simulink model "Simulation"  (R2016a)
settings: Solver=FixedStepAuto  StartTime=0.0  StopTime=20  FixedStep=0.01  RelTol=1e-3
undefined symbols (not defined in the file or in its folder): beta, g0, g1, g2, g3, gamma, kappa, landa, nu
(part 29 of 30)

== matlab function Simulation/U ==
  data: Ueq input; Uas input; u1 output; theta input; thetadot input; u2 output; u3 output; u4 output; u5 output; u6 output
function [u1,u2,u3,u4,u5,u6] = fcn(Ueq,Uas,theta,thetadot)


theta1=theta(1)
theta2=theta(2)
theta3=theta(3)
theta4=theta(4)
theta5=theta(5)
theta6=theta(6)

thetadot1=thetadot(1)
thetadot2=thetadot(2)
thetadot3=thetadot(3)
thetadot4=thetadot(4)
thetadot5=thetadot(5)
thetadot6=thetadot(6)
MM=[ 0.1*cos(theta2 + theta3)^2 + (0.1*cos(theta2)*cos(theta3)*cos(theta6)*sin(theta4) - 0.1*cos(theta6)*sin(theta2)*sin(theta3)*sin(theta4) + 0.1*cos(theta2)*sin(theta3)*sin(theta5)*sin(theta6) + 0.1*cos(theta3)*sin(theta2)*sin(theta5)*sin(theta6) - 0.1*cos(theta2)*cos(theta3)*cos(theta4)*cos(theta5)*sin(theta6) + 0.1*cos(theta4)*cos(theta5)*sin(theta2)*sin(theta3)*sin(theta6))*(cos(theta2)*cos(theta3)*cos(theta6)*sin(theta4) - 1.0*cos(theta6)*sin(theta2)*sin(theta3)*sin(theta4) + cos(theta2)*sin(theta3)*sin(theta5)*sin(theta6) + cos(theta3)*sin(theta2)*sin(theta5)*sin(theta6) - 1.0*cos(theta2)*cos(theta3)*cos(theta4)*cos(theta5)*sin(theta6) + cos(theta4)*cos(theta5)*sin(theta2)*sin(theta3)*sin(theta6)) + 0.2*sin(theta2 + theta3)^2 + (0.2*cos(theta2)*sin(theta4)*sin(theta5) + 0.4*sin(theta2)*sin(theta3)*sin(theta4) - 0.4*cos(theta2)*cos(theta3)*sin(theta4) + 0.4*cos(theta2)*cos(theta3)*cos(theta6)*sin(theta4) + 0.4*cos(theta2)*cos(theta3)*sin(theta4)*sin(theta5) - 0.4*cos(theta6)*sin(theta2)*sin(theta3)*sin(theta4) + 0.4*cos(theta2)*sin(theta3)*sin(theta5)*sin(theta6) + 0.4*cos(theta3)*sin(theta2)*sin(theta5)*sin(theta6) - 0.4*sin(theta2)*sin(theta3)*sin(theta4)*sin(theta5) - 0.4*cos(theta2)*cos(theta3)*cos(theta4)*cos(theta5)*sin(theta6) + 0.4*cos(theta4)*cos(theta5)*sin(theta2)*sin(theta3)*sin(theta6))^2 + 0.14*cos(theta2)^2 + 0.1*sin(theta2)^2 + (cos(theta2)*sin(theta3)*sin(theta5) + cos(theta3)*sin(theta2)*sin(theta5) - 1.0*cos(theta2)*cos(theta3)*cos(theta4)*cos(theta5) + cos(theta4)*cos(theta5)*sin(theta2)*sin(theta3))*(0.1*cos(theta2)*sin(theta3)*sin(theta5) + 0.1*cos(theta3)*sin(theta2)*sin(theta5) - 0.1*cos(theta2)*cos(theta3)*cos(theta4)*cos(theta5) + 0.1*cos(theta4)*cos(theta5)*sin(theta2)*sin(theta3)) + 2.0*(cos(theta2)*cos(theta5)*sin(theta3) + cos(theta3)*cos(theta5)*sin(theta2) + cos(theta2)*cos(theta3)*cos(theta4)*sin(theta5) - 1.0*cos(theta4)*sin(theta2)*sin(theta3)*sin(theta5))*(0.1*cos(theta2)*cos(theta5)*sin(theta3) + 0.1*cos(theta3)*cos(theta5)*sin(theta2) + 0.1*cos(theta2)*cos(theta3)*cos(theta4)*sin(theta5) - 0.1*cos(theta4)*sin(theta2)*sin(theta3)*sin(theta5)) + 0.04*cos(theta4)^2*(2.0*cos(theta2 + theta3) + cos(theta2))^2 + 0.1*cos(theta2 + theta3)^2*cos(theta4)^2 + 0.2*cos(theta2 + theta3)^2*sin(theta4)^2 + (0.1*cos(theta2)*cos(theta6)*sin(theta3)*sin(theta5) - 0.1*cos(theta2)*cos(theta3)*sin(theta4)*sin(theta6) + 0.1*cos(theta3)*cos(theta6)*sin(theta2)*sin(theta5) + 0.1*sin(theta2)*sin(theta3)*sin(theta4)*sin(theta6) - 0.1*cos(theta2)*cos(theta3)*cos(theta4)*cos(theta5)*cos(theta6) + 0.1*cos(theta4)*cos(theta5)*cos(theta6)*sin(theta2)*sin(theta3))*(cos(theta2)*cos(theta6)*sin(theta3)*sin(theta5) - 1.0*cos(theta2)*cos(theta3)*sin(theta4)*sin(theta6) + cos(theta3)*cos(theta6)*sin(theta2)*sin(theta5) + sin(theta2)*sin(theta3)*sin(theta4)*sin(theta6) - 1.0*cos(theta2)*cos(theta3)*cos(theta4)*cos(theta5)*cos(theta6) + cos(theta4)*cos(theta5)*cos(theta6)*sin(theta2)*sin(theta3)) + 0.04*cos(theta4)^2*(cos(theta2 + theta3) + cos(theta2))^2 + 0.04*sin(theta4)^2*(cos(theta2 + theta3) + cos(theta2))^2 + (0.2*cos(theta2)*cos(theta5)*cos(theta6)*sin(theta4) - 0.4*cos(theta2)*cos(theta3)*cos(theta4)*sin(theta6) - 0.2*cos(theta2)*cos(theta4)*sin(theta6) + 0.4*cos(theta2)*cos(theta5)*sin(theta3)*sin(theta6) + 0.4*cos(theta3)*cos(theta5)*sin(theta2)*sin(theta6) + 0.4*cos(theta4)*sin(theta2)*sin(theta3)*sin(theta6) + 0.4*cos(theta2)*cos(theta3)*cos(theta5)*cos(theta6)*sin(theta4) + 0.4*cos(theta2)*cos(theta3)*cos(theta4)*sin(theta5)*sin(theta6) - 0.4*cos(theta5)*cos(theta6)*sin(theta2)*sin(theta3)*sin(theta4) - 0.4*cos(theta4)*sin(theta2)*sin(theta3)*sin(theta5)*sin(theta6))^2 + (0.2*cos(theta2)*cos(theta4)*cos(theta6) + 0.4*cos(theta2)*cos(theta5)*sin(theta3) + 0.4*cos(theta3)*cos(theta5)*sin(theta2) + 0.4*cos(theta2)*cos(theta3)*cos(theta4)*cos(theta6) + 0.4*cos(theta2)*cos(theta3)*cos(theta4)*sin(theta5) - 0.4*cos(theta2)*cos(theta5)*cos(theta6)*sin(theta3) - 0.4*cos(theta3)*cos(theta5)*cos(theta6)*sin(theta2) - 0.4*cos(theta4)*cos(theta6)*sin(theta2)*sin(theta3) + 0.2*cos(theta2)*cos(theta5)*sin(theta4)*sin(theta6) - 0.4*cos(theta4)*sin(theta2)*sin(theta3)*sin(theta5) - 0.4*cos(theta2)*cos(theta3)*cos(theta4)*cos(theta6)*sin(theta5) + 0.4*cos(theta2)*cos(theta3)*cos(theta5)*sin(theta4)*sin(theta6) + 0.4*cos(theta4)*cos(theta6)*sin(theta2)*sin(theta3)*sin(theta5) - 0.4*cos(theta5)*sin(theta2)*sin(theta3)*sin(theta4)*sin(theta6))^2 + 0.04*cos(theta5)^2*sin(theta4)^2*(2.0*cos(theta2 + theta3) + cos(theta2))^2 + 0.04*sin(theta4)^2*sin(theta5)^2*(2.0*cos(theta2 + theta3) + cos(theta2))^2 + 0.1, 0.16*cos(theta2)*cos(theta3)*cos(theta4)*sin(theta4) - 0.08*cos(theta4)*sin(theta2)*sin(theta6) - 0.08*cos(theta5)*sin(theta2)*sin(theta4) + 0.16*cos(theta2)*cos(theta3)*cos(theta5)*sin(theta6) - 0.16*cos(theta2)*cos(theta5)*sin(theta3)*sin(theta4) - 0.16*cos(theta3)*cos(theta5)*sin(theta2)*sin(theta4) - 0.16*cos(theta2)*cos(theta4)*sin(theta3)*sin(theta6) - 0.16*cos(theta3)*cos(theta4)*sin(theta2)*sin(theta6) + 0.08*cos(theta5)*cos(theta6)*sin(theta2)*sin(theta4) - 0.16*cos(theta4)*sin(theta2)*sin(theta3)*sin(theta4) - 0.16*cos(theta5)*sin(theta2)*sin(theta3)*sin(theta6) - 0.16*cos(theta2)*cos(theta3)*cos(theta4)*cos(theta5)^2*sin(theta4) - 0.16*cos(theta2)*cos(theta3)*cos(theta4)*cos(theta6)^2*sin(theta4) - 0.32*cos(theta2)*cos(theta3)*cos(theta4)^2*cos(theta5)*sin(theta6) + 0.16*cos(theta4)*cos(theta5)^2*sin(theta2)*sin(theta3)*sin(theta4) + 0.16*cos(theta4)*cos(theta6)^2*sin(theta2)*sin(theta3)*sin(theta4) + 0.32*cos(theta4)^2*cos(theta5)*sin(theta2)*sin(theta3)*sin(theta6) - 0.16*cos(theta2)*cos(theta3)*cos(theta5)*cos(theta6)*sin(theta6) + 0.16*cos(theta2)*cos(theta5)*cos(theta6)*sin(theta3)*sin(theta4) + 0.16*cos(theta3)*cos(theta5)*cos(theta6)*sin(theta2)*sin(theta4) + 0.16*cos(theta2)*cos(theta5)*sin(theta3)*sin(theta4)*sin(theta5) + 0.16*cos(theta3)*cos(theta5)*sin(theta2)*sin(theta4)*sin(theta5) + 0.16*cos(theta2)*cos(theta4)*sin(theta3)*sin(theta5)*sin(theta6) + 0.16*cos(theta3)*cos(theta4)*sin(theta2)*sin(theta5)*sin(theta6) + 0.16*cos(theta5)*cos(theta6)*sin(theta2)*sin(theta3)*sin(theta6) - 0.16*cos(theta2)*cos(theta3)*cos(theta4)*cos(theta5)^2*cos(theta6)^2*sin(theta4) + 0.16*cos(theta4)*cos(theta5)^2*cos(theta6)^2*sin(theta2)*sin(theta3)*sin(theta4) - 0.32*cos(theta2)*cos(theta5)*cos(theta6)*sin(theta3)*sin(theta4)*sin(theta5) - 0.32*cos(theta3)*cos(theta5)*cos(theta6)*sin(theta2)*sin(theta4)*sin(theta5) - 0.16*cos(theta2)*cos(theta4)*cos(theta6)*sin(theta3)*sin(theta5)*sin(theta6) - 0.16*cos(theta3)*cos(theta4)*cos(theta6)*sin(theta2)*sin(theta5)*sin(theta6) + 0.32*cos(theta2)*cos(theta3)*cos(theta4)*cos(theta5)^2*cos(theta6)*sin(theta4) + 0.32*cos(theta2)*cos(theta3)*cos(theta4)^2*cos(theta5)*cos(theta6)*sin(theta6) - 0.32*cos(theta4)*cos(theta5)^2*cos(theta6)*sin(theta2)*sin(theta3)*sin(theta4) + 0.16*cos(theta2)*cos(theta5)*cos(theta6)^2*sin(theta3)*sin(theta4)*sin(theta5) + 0.16*cos(theta3)*cos(theta5)*cos(theta6)^2*sin(theta2)*sin(theta4)*sin(theta5) - 0.32*cos(theta4)^2*cos(theta5)*cos(theta6)*sin(theta2)*sin(theta3)*sin(theta6), 0.16*cos(theta2)*cos(theta3)*cos(theta4)*sin(theta4) + 0.16*cos(theta2)*cos(theta3)*cos(theta5)*sin(theta6) - 0.16*cos(theta2)*cos(theta5)*sin(theta3)*sin(theta4) - 0.16*cos(theta3)*cos(theta5)*sin(theta2)*sin(theta4) - 0.16*cos(theta2)*cos(theta4)*sin(theta3)*sin(theta6) - 0.16*cos(theta3)*cos(theta4)*sin(theta2)*sin(theta6) - 0.16*cos(theta4)*sin(theta2)*sin(theta3)*sin(theta4) - 0.16*cos(theta5)*sin(theta2)*sin(theta3)*sin(theta6) - 0.16*cos(theta2)*cos(theta3)*cos(theta4)*cos(theta5)^2*sin(theta4) - 0.16*cos(theta2)*cos(theta3)*cos(theta4)*cos(theta6)^2*sin(theta4) - 0.32*cos(theta2)*cos(theta3)*cos(theta4)^2*cos(theta5)*sin(theta6) + 0.16*cos(theta4)*cos(theta5)^2*sin(theta2)*sin(theta3)*sin(theta4) + 0.16*cos(theta4)*cos(theta6)^2*sin(theta2)*sin(theta3)*sin(theta4) + 0.32*cos(theta4)^2*cos(theta5)*sin(theta2)*sin(theta3)*sin(theta6) - 0.16*cos(theta2)*cos(theta3)*cos(theta5)*cos(theta6)*sin(theta6) + 0.16*cos(theta2)*cos(theta5)*cos(theta6)*sin(theta3)*sin(theta4) + 0.16*cos(theta3)*cos(theta5)*cos(theta6)*sin(theta2)*sin(theta4) + 0.16*cos(theta2)*cos(theta5)*sin(theta3)*sin(theta4)*sin(theta5) + 0.16*cos(theta3)*cos(theta5)*sin(theta2)*sin(theta4)*sin(theta5) + 0.16*cos(theta2)*cos(theta4)*sin(theta3)*sin(theta5)*sin(theta6) + 0.16*cos(theta3)*cos(theta4)*sin(theta2)*sin(theta5)*sin(theta6) + 0.16*cos(theta5)*cos(theta6)*sin(theta2)*sin(theta3)*sin(theta6) - 0.16*cos(theta2)*cos(theta3)*cos(theta4)*cos(theta5)^2*cos(theta6)^2*sin(theta4) + 0.16*cos(theta4)*cos(theta5)^2*cos(theta6)^2*sin(theta2)*sin(theta3)*sin(theta4) - 0.32*cos(theta2)*cos(theta5)*cos(theta6)*sin(theta3)*sin(theta4)*sin(theta5) - 0.32*cos(theta3)*cos(theta5)*cos(theta6)*sin(theta2)*sin(theta4)*sin(theta5) - 0.16*cos(theta2)*cos(theta4)*cos(theta6)*sin(theta3)*sin(theta5)*sin(theta6) - 0.16*cos(theta3)*cos(theta4)*cos(theta6)*sin(theta2)*sin(theta5)*sin(theta6) + 0.32*cos(theta2)*cos(theta3)*cos(theta4)*cos(theta5)^2*cos(theta6)*sin(theta4) + 0.32*cos(theta2)*cos(theta3)*cos(theta4)^2*cos(theta5)*cos(theta6)*sin(theta6) - 0.32*cos(theta4)*cos(theta5)^2*cos(theta6)*sin(theta2)*sin(theta3)*sin(theta4) + 0.16*cos(theta2)*cos(theta5)*cos(theta6)^2*sin(theta3)*sin(theta4)*sin(theta5) + 0.16*cos(theta3)*cos(theta5)*cos(theta6)^2*sin(theta2)*sin(theta4)*sin(theta5) - 0.32*cos(theta4)^2*cos(theta5)*cos(theta6)*sin(theta2)*sin(theta3)*sin(theta6), 0.46*cos(theta2)*sin(theta3) + 0.46*cos(theta3)*sin(theta2) + 0.08*cos(theta2)*sin(theta4)*sin(theta6) + 0.16*cos(theta2)*cos(theta5)^2*sin(theta3) + 0.16*cos(theta3)*cos(theta5)^2*sin(theta2) - 0.16*cos(theta2)*cos(theta6)^2*sin(theta3) - 0.16*cos(theta3)*cos(theta6)^2*sin(theta2) - 0.08*cos(theta2)*cos(theta4)*cos(theta5) - 0.32*cos(theta2)*cos(theta5)^2*cos(theta6)*sin(theta3) - 0.32*cos(theta3)*cos(theta5)^2*cos(theta6)*sin(theta2) + 0.16*cos(theta2)*cos(theta5)^2*cos(theta6)^2*sin(theta3) + 0.16*cos(theta3)*cos(theta5)^2*cos(theta6)^2*sin(theta2) - 0.16*cos(theta2)*cos(theta3)*cos(theta4)*cos(theta5) + 0.08*cos(theta2)*cos(theta4)*cos(theta5)*cos(theta6) + 0.16*cos(theta4)*cos(theta5)*sin(theta2)*sin(theta3) + 0.16*cos(theta2)*cos(theta3)*sin(theta4)*sin(theta6) - 0.16*sin(theta2)*sin(theta3)*sin(theta4)*sin(theta6) + 0.16*cos(theta2)*cos(theta3)*cos(theta4)*cos(theta5)*cos(theta6) + 0.16*cos(theta2)*cos(theta3)*cos(theta4)*cos(theta5)*sin(theta5) - 0.16*cos(theta4)*cos(theta5)*cos(theta6)*sin(theta2)*sin(theta3) - 0.16*cos(theta4)*cos(theta5)*sin(theta2)*sin(theta3)*sin(theta5) - 0.16*cos(theta2)*cos(theta3)*sin(theta4)*sin(theta5)*sin(theta6) + 0.16*sin(theta2)*sin(theta3)*sin(theta4)*sin(theta5)*sin(theta6) - 0.32*cos(theta2)*cos(theta3)*cos(theta4)*cos(theta5)*cos(theta6)*sin(theta5) + 0.32*cos(theta4)*cos(theta5)*cos(theta6)*sin(theta2)*sin(theta3)*sin(theta5) + 0.16*cos(theta2)*cos(theta3)*cos(theta6)*sin(theta4)*sin(theta5)*sin(theta6) - 0.16*cos(theta6)*sin(theta2)*sin(theta3)*sin(theta4)*sin(theta5)*sin(theta6) + 0.16*cos(theta2)*cos(theta3)*cos(theta4)*cos(theta5)*cos(theta6)^2*sin(theta5) - 0.16*cos(theta4)*cos(theta5)*cos(theta6)^2*sin(theta2)*sin(theta3)*sin(theta5), 0.08*cos(theta2)*sin(theta4)*sin(theta5) + 0.36*sin(theta2)*sin(theta3)*sin(theta4) - 0.36*cos(theta2)*cos(theta3)*sin(theta4) - 0.16*cos(theta2)*cos(theta3)*cos(theta6)^2*sin(theta4) + 0.16*cos(theta6)^2*sin(theta2)*sin(theta3)*sin(theta4) + 0.32*cos(theta2)*cos(theta3)*cos(theta6)*sin(theta4) + 0.16*cos(theta2)*cos(theta3)*sin(theta4)*sin(theta5) - 0.08*cos(theta2)*cos(theta6)*sin(theta4)*sin(theta5) - 0.32*cos(theta6)*sin(theta2)*sin(theta3)*sin(theta4) + 0.16*cos(theta2)*sin(theta3)*sin(theta5)*sin(theta6) + 0.16*cos(theta3)*sin(theta2)*sin(theta5)*sin(theta6) - 0.16*sin(theta2)*sin(theta3)*sin(theta4)*sin(theta5) - 0.16*cos(theta2)*cos(theta3)*cos(theta4)*cos(theta5)*sin(theta6) - 0.16*cos(theta2)*cos(theta3)*cos(theta6)*sin(theta4)*sin(theta5) + 0.16*cos(theta4)*cos(theta5)*sin(theta2)*sin(theta3)*sin(theta6) - 0.16*cos(theta2)*cos(theta6)*sin(theta3)*sin(theta5)*sin(theta6) - 0.16*cos(theta3)*cos(theta6)*sin(theta2)*sin(theta5)*sin(theta6) + 0.16*cos(theta6)*sin(theta2)*sin(theta3)*sin(theta4)*sin(theta5) + 0.16*cos(theta2)*cos(theta3)*cos(theta4)*cos(theta5)*cos(theta6)*sin(theta6) - 0.16*cos(theta4)*cos(theta5)*cos(theta6)*sin(theta2)*sin(theta3)*sin(theta6), 0.08*cos(theta2)*cos(theta4)*cos(theta6) + 0.26*cos(theta2)*cos(theta5)*sin(theta3) + 0.26*cos(theta3)*cos(theta5)*sin(theta2) + 0.16*cos(theta2)*cos(theta3)*cos(theta4)*cos(theta6) + 0.26*cos(theta2)*cos(theta3)*cos(theta4)*sin(theta5) - 0.16*cos(theta2)*cos(theta5)*cos(theta6)*sin(theta3) - 0.16*cos(theta3)*cos(theta5)*cos(theta6)*sin(theta2) - 0.16*cos(theta4)*cos(theta6)*sin(theta2)*sin(theta3) + 0.08*cos(theta2)*cos(theta5)*sin(theta4)*sin(theta6) - 0.26*cos(theta4)*sin(theta2)*sin(theta3)*sin(theta5) - 0.16*cos(theta2)*cos(theta3)*cos(theta4)*cos(theta6)*sin(theta5) + 0.16*cos(theta2)*cos(theta3)*cos(theta5)*sin(theta4)*sin(theta6) + 0.16*cos(theta4)*cos(theta6)*sin(theta2)*sin(theta3)*sin(theta5) - 0.16*cos(theta5)*sin(theta2)*sin(theta3)*sin(theta4)*sin(theta6);
                                                                                                                                                                                                                                                                                                                                                                                                                                                                                                                                                                                                                                                                                                                                                                                                                                                                                                                                                                                                                                                                                                                                                                                                                                                                                                                                                                                                                                                                                                                                                                                                                                                                                                                                                                                                                                                                                                                                                                                                                                                                                                                                                                       0.16*cos(theta2)*cos(theta3)*cos(theta4)*sin(theta4) - 0.08*cos(theta4)*sin(theta2)*sin(theta6) - 0.08*cos(theta5)*sin(theta2)*sin(theta4) + 0.16*cos(theta2)*cos(theta3)*cos(theta5)*sin(theta6) - 0.16*cos(theta2)*cos(theta5)*sin(theta3)*sin(theta4) - 0.16*cos(theta3)*cos(theta5)*sin(theta2)*sin(theta4) - 0.16*cos(theta2)*cos(theta4)*sin(theta3)*sin(theta6) - 0.16*cos(theta3)*cos(theta4)*sin(theta2)*sin(theta6) + 0.08*cos(theta5)*cos(theta6)*sin(theta2)*sin(theta4) - 0.16*cos(theta4)*sin(theta2)*sin(theta3)*sin(theta4) - 0.16*cos(theta5)*sin(theta2)*sin(theta3)*sin(theta6) - 0.16*cos(theta2)*cos(theta3)*cos(theta4)*cos(theta5)^2*sin(theta4) - 0.16*cos(theta2)*cos(theta3)*cos(theta4)*cos(theta6)^2*sin(theta4) - 0.32*cos(theta2)*cos(theta3)*cos(theta4)^2*cos(theta5)*sin(theta6) + 0.16*cos(theta4)*cos(theta5)^2*sin(theta2)*sin(theta3)*sin(theta4) + 0.16*cos(theta4)*cos(theta6)^2*sin(theta2)*sin(theta3)*sin(theta4) + 0.32*cos(theta4)^2*cos(theta5)*sin(theta2)*sin(theta3)*sin(theta6) - 0.16*cos(theta2)*cos(theta3)*cos(theta5)*cos(theta6)*sin(theta6) + 0.16*cos(theta2)*cos(theta5)*cos(theta6)*sin(theta3)*sin(theta4) + 0.16*cos(theta3)*cos(theta5)*cos(theta6)*sin(theta2)*sin(theta4) + 0.16*cos(theta2)*cos(theta5)*sin(theta3)*sin(theta4)*sin(theta5) + 0.16*cos(theta3)*cos(theta5)*sin(theta2)*sin(theta4)*sin(theta5) + 0.16*cos(theta2)*cos(theta4)*sin(theta3)*sin(theta5)*sin(theta6) + 0.16*cos(theta3)*cos(theta4)*sin(theta2)*sin(theta5)*sin(theta6) + 0.16*cos(theta5)*cos(theta6)*sin(theta2)*sin(theta3)*sin(theta6) - 0.16*cos(theta2)*cos(theta3)*cos(theta4)*cos(theta5)^2*cos(theta6)^2*sin(theta4) + 0.16*cos(theta4)*cos(theta5)^2*cos(theta6)^2*sin(theta2)*sin(theta3)*sin(theta4) - 0.32*cos(theta2)*cos(theta5)*cos(theta6)*sin(theta3)*sin(theta4)*sin(theta5) - 0.32*cos(theta3)*cos(theta5)*cos(theta6)*sin(theta2)*sin(theta4)*sin(theta5) - 0.16*cos(theta2)*cos(theta4)*cos(theta6)*sin(theta3)*sin(theta5)*sin(theta6) - 0.16*cos(theta3)*cos(theta4)*cos(theta6)*sin(theta2)*sin(theta5)*sin(theta6) + 0.32*cos(theta2)*cos(theta3)*cos(theta4)*cos(theta5)^2*cos(theta6)*sin(theta4) + 0.32*cos(theta2)*cos(theta3)*cos(theta4)^2*cos(theta5)*cos(theta6)*sin(theta6) - 0.32*cos(theta4)*cos(theta5)^2*cos(theta6)*sin(theta2)*sin(theta3)*sin(theta4) + 0.16*cos(theta2)*cos(theta5)*cos(theta6)^2*sin(theta3)*sin(theta4)*sin(theta5) + 0.16*cos(theta3)*cos(theta5)*cos(theta6)^2*sin(theta2)*sin(theta4)*sin(theta5) - 0.32*cos(theta4)^2*cos(theta5)*cos(theta6)*sin(theta2)*sin(theta3)*sin(theta6),                                                                                                                                                                                                                                                                                                                                                                                                                                                                                                                                                                                                                                                                                                                                                                                                                                                                                                                                                                                                                         (0.1*cos(theta4)*cos(theta6) + 0.1*cos(theta5)*sin(theta4)*sin(theta6))*(cos(theta4)*cos(theta6) + cos(theta5)*sin(theta4)*sin(theta6)) + (0.4*cos(theta4)*cos(theta5) - 0.2*sin(theta3)*sin(theta5) + 0.2*cos(theta3)*cos(theta4)*cos(theta5))^2 + (0.4*sin(theta4)*sin(theta6) + 0.2*cos(theta3)*sin(theta4)*sin(theta6) - 0.2*cos(theta6)*sin(theta3)*sin(theta5) - 0.4*sin(theta4)*sin(theta5)*sin(theta6) + 0.4*cos(theta4)*cos(theta5)*cos(theta6) + 0.2*cos(theta3)*cos(theta4)*cos(theta5)*cos(theta6))^2 + (0.2*cos(theta5)*sin(theta3) + 0.4*cos(theta4)*sin(theta5) + 0.2*cos(theta3)*cos(theta4)*sin(theta5))^2 + 0.04*cos(theta3)^2 + 0.2*cos(theta4)^2 + 0.08*sin(theta3)^2 + 0.1*sin(theta4)^2 + (0.1*cos(theta4)*sin(theta6) - 0.1*cos(theta5)*cos(theta6)*sin(theta4))*(cos(theta4)*sin(theta6) - 1.0*cos(theta5)*cos(theta6)*sin(theta4)) + 0.04*cos(theta4)^2*(cos(theta3) + 1.0)^2 + 0.04*sin(theta4)^2*(cos(theta3) + 1.0)^2 + 0.04*sin(theta4)^2*(cos(theta3) + 2.0)^2 + (0.4*cos(theta4)*cos(theta6) - 0.4*cos(theta4) + 0.2*cos(theta5)*sin(theta3) + 0.4*cos(theta4)*sin(theta5) + 0.4*cos(theta5)*sin(theta4)*sin(theta6) + 0.2*cos(theta3)*cos(theta4)*sin(theta5))^2 + (0.4*cos(theta6)*sin(theta4) + 0.4*sin(theta4)*sin(theta5) - 0.4*cos(theta6)*sin(theta4)*sin(theta5) + 0.2*sin(theta3)*sin(theta5)*sin(theta6) + 0.2*cos(theta3)*cos(theta6)*sin(theta4) - 0.4*cos(theta4)*cos(theta5)*sin(theta6) - 0.2*cos(theta3)*cos(theta4)*cos(theta5)*sin(theta6))^2 + 0.1*cos(theta5)^2*sin(theta4)^2 + 0.2*sin(theta4)^2*sin(theta5)^2 + 0.2,                                                                                                                                                                                                                                                                                                                                                                                                                                                                                                                                                                                                                                                                                                                                                                                                                                                                                                                                                                                                                                                                                                                                                                                                                                                                                                                                                                                                                                                                                                                                                                                                                                                                                                                    0.2*cos(theta3) - 0.32*cos(theta6) - 0.32*sin(theta5) - 0.08*cos(theta3)*sin(theta5) + 0.32*cos(theta6)*sin(theta5) - 0.16*cos(theta4)^2 - 0.16*cos(theta5)^2 + 0.32*cos(theta5)^2*cos(theta6) + 0.16*cos(theta4)^2*cos(theta5)^2 + 0.16*cos(theta4)^2*cos(theta6)^2 - 0.16*cos(theta5)^2*cos(theta6)^2 + 0.16*cos(theta4)^2*cos(theta5)^2*cos(theta6)^2 + 0.08*sin(theta3)*sin(theta4)*sin(theta6) - 0.32*cos(theta4)^2*cos(theta5)^2*cos(theta6) - 0.08*cos(theta4)*cos(theta5)*sin(theta3) + 0.08*cos(theta3)*cos(theta6)*sin(theta5) + 0.08*cos(theta4)*cos(theta5)*cos(theta6)*sin(theta3) - 0.32*cos(theta4)*cos(theta5)*sin(theta4)*sin(theta6) + 0.32*cos(theta4)*cos(theta5)*cos(theta6)*sin(theta4)*sin(theta6) + 1.08,                                                                                                                                                                                                                                                                                                                                                                                                                                                                                                                                                                                                                                                                                                                                                                                                                                                                                                                                                                                                                                                                                                                                                                                                                                                                                                                                                                                                                                                                                                                                                                                                        -(2*(cos(theta5)*sin(theta4) + cos(theta4)*sin(theta6) - 1.0*cos(theta5)*cos(theta6)*sin(theta4))*(cos(theta3) - 2.0*sin(theta5) + 2.0*cos(theta6)*sin(theta5) + 2.0))/25,                                                                                                                                                                                                                                                                                                                                                                                                                                                                                                                                                                                                                                                                                                                                                                                                             0.1*cos(theta4) + (0.4*cos(theta6) - 0.4)*(0.4*cos(theta4)*cos(theta6) - 0.4*cos(theta4) + 0.2*cos(theta5)*sin(theta3) + 0.4*cos(theta4)*sin(theta5) + 0.4*cos(theta5)*sin(theta4)*sin(theta6) + 0.2*cos(theta3)*cos(theta4)*sin(theta5)) + cos(theta6)*(0.1*cos(theta4)*cos(theta6) + 0.1*cos(theta5)*sin(theta4)*sin(theta6)) + sin(theta6)*(0.1*cos(theta4)*sin(theta6) - 0.1*cos(theta5)*cos(theta6)*sin(theta4)),                                                                                                                                                                                                                                                                                                                                                                                                                                                                                                              0.16*cos(theta6)*sin(theta4) + 0.26*sin(theta4)*sin(theta5) - 0.16*cos(theta6)*sin(theta4)*sin(theta5) + 0.08*sin(theta3)*sin(theta5)*sin(theta6) + 0.08*cos(theta3)*cos(theta6)*sin(theta4) - 0.16*cos(theta4)*cos(theta5)*sin(theta6) - 0.08*cos(theta3)*cos(theta4)*cos(theta5)*sin(theta6);
                                                                                                                                                                                                                                                                                                                                                                                                                                                                                                                                                                                                                                                                                                                                                                                                                                                                                                                                                                                                                                                                                                                                                                                                                                                                                                                                                                                                                                                                                                                                                                                                                                                                                                                                                                                                                                                                                                                                                                                                                                                                                                                                                                                                                                                                                                                   0.16*cos(theta2)*cos(theta3)*cos(theta4)*sin(theta4) + 0.16*cos(theta2)*cos(theta3)*cos(theta5)*sin(theta6) - 0.16*cos(theta2)*cos(theta5)*sin(theta3)*sin(theta4) - 0.16*cos(theta3)*cos(theta5)*sin(theta2)*sin(theta4) - 0.16*cos(theta2)*cos(theta4)*sin(theta3)*sin(theta6) - 0.16*cos(theta3)*cos(theta4)*sin(theta2)*sin(theta6) - 0.16*cos(theta4)*sin(theta2)*sin(theta3)*sin(theta4) - 0.16*cos(theta5)*sin(theta2)*sin(theta3)*sin(theta6) - 0.16*cos(theta2)*cos(theta3)*cos(theta4)*cos(theta5)^2*sin(theta4) - 0.16*cos(theta2)*cos(theta3)*cos(theta4)*cos(theta6)^2*sin(theta4) - 0.32*cos(theta2)*cos(theta3)*cos(theta4)^2*cos(theta5)*sin(theta6) + 0.16*cos(theta4)*cos(theta5)^2*sin(theta2)*sin(theta3)*sin(theta4) + 0.16*cos(theta4)*cos(theta6)^2*sin(theta2)*sin(theta3)*sin(theta4) + 0.32*cos(theta4)^2*cos(theta5)*sin(theta2)*sin(theta3)*sin(theta6) - 0.16*cos(theta2)*cos(theta3)*cos(theta5)*cos(theta6)*sin(theta6) + 0.16*cos(theta2)*cos(theta5)*cos(theta6)*sin(theta3)*sin(theta4) + 0.16*cos(theta3)*cos(theta5)*cos(theta6)*sin(theta2)*sin(theta4) + 0.16*cos(theta2)*cos(theta5)*sin(theta3)*sin(theta4)*sin(theta5) + 0.16*cos(theta3)*cos(theta5)*sin(theta2)*sin(theta4)*sin(theta5) + 0.16*cos(theta2)*cos(theta4)*sin(theta3)*sin(theta5)*sin(theta6) + 0.16*cos(theta3)*cos(theta4)*sin(theta2)*sin(theta5)*sin(theta6) + 0.16*cos(theta5)*cos(theta6)*sin(theta2)*sin(theta3)*sin(theta6) - 0.16*cos(theta2)*cos(theta3)*cos(theta4)*cos(theta5)^2*cos(theta6)^2*sin(theta4) + 0.16*cos(theta4)*cos(theta5)^2*cos(theta6)^2*sin(theta2)*sin(theta3)*sin(theta4) - 0.32*cos(theta2)*cos(theta5)*cos(theta6)*sin(theta3)*sin(theta4)*sin(theta5) - 0.32*cos(theta3)*cos(theta5)*cos(theta6)*sin(theta2)*sin(theta4)*sin(theta5) - 0.16*cos(theta2)*cos(theta4)*cos(theta6)*sin(theta3)*sin(theta5)*sin(theta6) - 0.16*cos(theta3)*cos(theta4)*cos(theta6)*sin(theta2)*sin(theta5)*sin(theta6) + 0.32*cos(theta2)*cos(theta3)*cos(theta4)*cos(theta5)^2*cos(theta6)*sin(theta4) + 0.32*cos(theta2)*cos(theta3)*cos(theta4)^2*cos(theta5)*cos(theta6)*sin(theta6) - 0.32*cos(theta4)*cos(theta5)^2*cos(theta6)*sin(theta2)*sin(theta3)*sin(theta4) + 0.16*cos(theta2)*cos(theta5)*cos(theta6)^2*sin(theta3)*sin(theta4)*sin(theta5) + 0.16*cos(theta3)*cos(theta5)*cos(theta6)^2*sin(theta2)*sin(theta4)*sin(theta5) - 0.32*cos(theta4)^2*cos(theta5)*cos(theta6)*sin(theta2)*sin(theta3)*sin(theta6),                                                                                                                                                                                                                                                                                                                                                                                                                                                                                                                                                                                                                                                                                                                                                                                                                                                                                                                                                                                                                                                                                                                                                                                                                                                                                                                                                                                                                                                                                                                                                                                                                                                                                                                                                                                                                                                                 0.2*cos(theta3) - 0.32*cos(theta6) - 0.32*sin(theta5) - 0.08*cos(theta3)*sin(theta5) + 0.32*cos(theta6)*sin(theta5) - 0.16*cos(theta4)^2 - 0.16*cos(theta5)^2 + 0.32*cos(theta5)^2*cos(theta6) + 0.16*cos(theta4)^2*cos(theta5)^2 + 0.16*cos(theta4)^2*cos(theta6)^2 - 0.16*cos(theta5)^2*cos(theta6)^2 + 0.16*cos(theta4)^2*cos(theta5)^2*cos(theta6)^2 + 0.08*sin(theta3)*sin(theta4)*sin(theta6) - 0.32*cos(theta4)^2*cos(theta5)^2*cos(theta6) - 0.08*cos(theta4)*cos(theta5)*sin(theta3) + 0.08*cos(theta3)*cos(theta6)*sin(theta5) + 0.08*cos(theta4)*cos(theta5)*cos(theta6)*sin(theta3) - 0.32*cos(theta4)*cos(theta5)*sin(theta4)*sin(theta6) + 0.32*cos(theta4)*cos(theta5)*cos(theta6)*sin(theta4)*sin(theta6) + 1.08,                                                                                                                                                                                                                                                                                                                                                                                                                                                                                                                                                                                                                                                                                                                                                                                                                                                                                                                                                                                                                                                                                                                                                                                                                                                                                                                                                                                                                                                                                                                                                                (0.1*cos(theta4)*cos(theta6) + 0.1*cos(theta5)*sin(theta4)*sin(theta6))*(cos(theta4)*cos(theta6) + cos(theta5)*sin(theta4)*sin(theta6)) + (0.4*sin(theta4)*sin(theta6) - 0.4*sin(theta4)*sin(theta5)*sin(theta6) + 0.4*cos(theta4)*cos(theta5)*cos(theta6))^2 + 0.24*cos(theta4)^2 + 0.3*sin(theta4)^2 + (0.1*cos(theta4)*sin(theta6) - 0.1*cos(theta5)*cos(theta6)*sin(theta4))*(cos(theta4)*sin(theta6) - 1.0*cos(theta5)*cos(theta6)*sin(theta4)) + (0.4*cos(theta6)*sin(theta4) + 0.4*sin(theta4)*sin(theta5) - 0.4*cos(theta6)*sin(theta4)*sin(theta5) - 0.4*cos(theta4)*cos(theta5)*sin(theta6))^2 + (0.4*cos(theta4)*cos(theta6) - 0.4*cos(theta4) + 0.4*cos(theta4)*sin(theta5) + 0.4*cos(theta5)*sin(theta4)*sin(theta6))^2 + 0.16*cos(theta4)^2*cos(theta5)^2 + 0.16*cos(theta4)^2*sin(theta5)^2 + 0.1*cos(theta5)^2*sin(theta4)^2 + 0.2*sin(theta4)^2*sin(theta5)^2 + 0.1,                                                                                                                                                                                                                                                                                                                                                                                                                                                                                                                                                                                                                                                                                                                                                                                                                                                                                                                                                                                                                                                                                                                                                                                                                                                                                                                                                                                                                                                                                                                                                                                                                          -(4*(cos(theta6)*sin(theta5) - 1.0*sin(theta5) + 1.0)*(cos(theta5)*sin(theta4) + cos(theta4)*sin(theta6) - 1.0*cos(theta5)*cos(theta6)*sin(theta4)))/25,                                                                                                                                                                                                                                                                                                                                                                                                                                                                                                                                                                                                                                                                                                                                                                                                                                                                                                                                                                      0.36*cos(theta4) - 0.32*cos(theta4)*cos(theta6) - 0.16*cos(theta4)*sin(theta5) + 0.16*cos(theta4)*cos(theta6)^2 - 0.16*cos(theta5)*sin(theta4)*sin(theta6) + 0.16*cos(theta4)*cos(theta6)*sin(theta5) + 0.16*cos(theta5)*cos(theta6)*sin(theta4)*sin(theta6),                                                                                                                                                                                                                                                                                                                                                                                                                                                                                                                                                                                                                                                           0.16*cos(theta6)*sin(theta4) + 0.26*sin(theta4)*sin(theta5) - 0.16*cos(theta6)*sin(theta4)*sin(theta5) - 0.16*cos(theta4)*cos(theta5)*sin(theta6);
                                                                                                                                                                                                                                                                                                                                                                                                                                                                                                                                                                                                                                                                                                                                                                                                                                                                                                                                                                                                                                                                                                                                                                                                                                                                                                                                                                                                                                                                                                                                                                                                                                                                                                                                                                                                                                                                                                                                                                                                                                                                                                                                                                                                                                                                                                                                                                                                                                                                                                                                                                                                                                                                                                                                                                                                                                                                                                                                                                                       0.46*cos(theta2)*sin(theta3) + 0.46*cos(theta3)*sin(theta2) + 0.08*cos(theta2)*sin(theta4)*sin(theta6) + 0.16*cos(theta2)*cos(theta5)^2*sin(theta3) + 0.16*cos(theta3)*cos(theta5)^2*sin(theta2) - 0.16*cos(theta2)*cos(theta6)^2*sin(theta3) - 0.16*cos(theta3)*cos(theta6)^2*sin(theta2) - 0.08*cos(theta2)*cos(theta4)*cos(theta5) - 0.32*cos(theta2)*cos(theta5)^2*cos(theta6)*sin(theta3) - 0.32*cos(theta3)*cos(theta5)^2*cos(theta6)*sin(theta2) + 0.16*cos(theta2)*cos(theta5)^2*cos(theta6)^2*sin(theta3) + 0.16*cos(theta3)*cos(theta5)^2*cos(theta6)^2*sin(theta2) - 0.16*cos(theta2)*cos(theta3)*cos(theta4)*cos(theta5) + 0.08*cos(theta2)*cos(theta4)*cos(theta5)*cos(theta6) + 0.16*cos(theta4)*cos(theta5)*sin(theta2)*sin(theta3) + 0.16*cos(theta2)*cos(theta3)*sin(theta4)*sin(theta6) - 0.16*sin(theta2)*sin(theta3)*sin(theta4)*sin(theta6) + 0.16*cos(theta2)*cos(theta3)*cos(theta4)*cos(theta5)*cos(theta6) + 0.16*cos(theta2)*cos(theta3)*cos(theta4)*cos(theta5)*sin(theta5) - 0.16*cos(theta4)*cos(theta5)*cos(theta6)*sin(theta2)*sin(theta3) - 0.16*cos(theta4)*cos(theta5)*sin(theta2)*sin(theta3)*sin(theta5) - 0.16*cos(theta2)*cos(theta3)*sin(theta4)*sin(theta5)*sin(theta6) + 0.16*sin(theta2)*sin(theta3)*sin(theta4)*sin(theta5)*sin(theta6) - 0.32*cos(theta2)*cos(theta3)*cos(theta4)*cos(theta5)*cos(theta6)*sin(theta5) + 0.32*cos(theta4)*cos(theta5)*cos(theta6)*sin(theta2)*sin(theta3)*sin(theta5) + 0.16*cos(theta2)*cos(theta3)*cos(theta6)*sin(theta4)*sin(theta5)*sin(theta6) - 0.16*cos(theta6)*sin(theta2)*sin(theta3)*sin(theta4)*sin(theta5)*sin(theta6) + 0.16*cos(theta2)*cos(theta3)*cos(theta4)*cos(theta5)*cos(theta6)^2*sin(theta5) - 0.16*cos(theta4)*cos(theta5)*cos(theta6)^2*sin(theta2)*sin(theta3)*sin(theta5),                                                                                                                                                                                                                                                                                                                                                                                                                                                                                                                                                                                                                                                                                                                                                                                                                                                                                                                                                                                                                                                                                                                                                                                                                                                                                                                                                                                                                                                                                                                                                                                                                                                                                                                                                                                                                                                                                                                                                                                                                                                                                                                                                                                                                                                                                                                                                                                                                        -(2*(cos(theta5)*sin(theta4) + cos(theta4)*sin(theta6) - 1.0*cos(theta5)*cos(theta6)*sin(theta4))*(cos(theta3) - 2.0*sin(theta5) + 2.0*cos(theta6)*sin(theta5) + 2.0))/25,                                                                                                                                                                                                                                                                                                                                                                                                                                                                                                                                                                                                                                                                                                                                                                                                                                                                                                                                                                                                                                                                                                                                                                                                                                                                                                                                                                                                                                                                                                                                                                                                                                                                                                                                                                                                                                                                                                                                                                                                                                                                                                                                                                                                                                                                                             -(4*(cos(theta6)*sin(theta5) - 1.0*sin(theta5) + 1.0)*(cos(theta5)*sin(theta4) + cos(theta4)*sin(theta6) - 1.0*cos(theta5)*cos(theta6)*sin(theta4)))/25,                                                                                                                                                                                                                                                                                                                                                                                                                                                                                                                                                                                                                                                                                                                                                                                                                                                                                                                                                                                                                                                                                                                                                                                                                                                                                                                                                                                                                                                                                                                                                                                                                                                               0.16*cos(theta5)^2 - 0.16*cos(theta6)^2 - 0.32*cos(theta5)^2*cos(theta6) + 0.16*cos(theta5)^2*cos(theta6)^2 + 0.46,                                                                                                                                                                                                                                                                                                                                                                                                                                                                                                                                                                                                                                                                                                                                                                                                                                                                                                                                                                                                                                                                                                                                                                              -0.4*sin(theta5)*sin(theta6)*(0.4*cos(theta6) - 0.4),                                                                                                                                                                                                                                                                                                                                                                                                                                                                                                                                                                                                                                                                                                                                                                  -(cos(theta5)*(8.0*cos(theta6) - 13.0))/50;
                                                                                                                                                                                                                                                                                                                                                                                                                                                                                                                                                                                                                                                                                                                                                                                                                                                                                                                                                                                                                                                                                                                                                                                                                                                                                                                                                                                                                                                                                                                                                                                                                                                                                                                                                                                                                                                                                                                                                                                                                                                                                                                                                                                                                                                                                                                                                                                                                                                                                                                                                                                                                                                                                                                                                                                                                                                                                                                                                                                                                                                                                                                                                                                                                                                                                                                                                                                                                                                                                                                                      0.08*cos(theta2)*sin(theta4)*sin(theta5) + 0.36*sin(theta2)*sin(theta3)*sin(theta4) - 0.36*cos(theta2)*cos(theta3)*sin(theta4) - 0.16*cos(theta2)*cos(theta3)*cos(theta6)^2*sin(theta4) + 0.16*cos(theta6)^2*sin(theta2)*sin(theta3)*sin(theta4) + 0.32*cos(theta2)*cos(theta3)*cos(theta6)*sin(theta4) + 0.16*cos(theta2)*cos(theta3)*sin(theta4)*sin(theta5) - 0.08*cos(theta2)*cos(theta6)*sin(theta4)*sin(theta5) - 0.32*cos(theta6)*sin(theta2)*sin(theta3)*sin(theta4) + 0.16*cos(theta2)*sin(theta3)*sin(theta5)*sin(theta6) + 0.16*cos(theta3)*sin(theta2)*sin(theta5)*sin(theta6) - 0.16*sin(theta2)*sin(theta3)*sin(theta4)*sin(theta5) - 0.16*cos(theta2)*cos(theta3)*cos(theta4)*cos(theta5)*sin(theta6) - 0.16*cos(theta2)*cos(theta3)*cos(theta6)*sin(theta4)*sin(theta5) + 0.16*cos(theta4)*cos(theta5)*sin(theta2)*sin(theta3)*sin(theta6) - 0.16*cos(theta2)*cos(theta6)*sin(theta3)*sin(theta5)*sin(theta6) - 0.16*cos(theta3)*cos(theta6)*sin(theta2)*sin(theta5)*sin(theta6) + 0.16*cos(theta6)*sin(theta2)*sin(theta3)*sin(theta4)*sin(theta5) + 0.16*cos(theta2)*cos(theta3)*cos(theta4)*cos(theta5)*cos(theta6)*sin(theta6) - 0.16*cos(theta4)*cos(theta5)*cos(theta6)*sin(theta2)*sin(theta3)*sin(theta6),                                                                                                                                                                                                                                                                                                                                                                                                                                                                                                                                                                                                                                                                                                                                                                                                                                                                                                                                                                                                                                                                                                                                                                                                                                                                                                                                                                                                                                                                                                                                                                                                                                                                                                                                                                                                                                                                                                                                                                                                                                                                                                                                                                                0.1*cos(theta4) + (0.4*cos(theta6) - 0.4)*(0.4*cos(theta4)*cos(theta6) - 0.4*cos(theta4) + 0.2*cos(theta5)*sin(theta3) + 0.4*cos(theta4)*sin(theta5) + 0.4*cos(theta5)*sin(theta4)*sin(theta6) + 0.2*cos(theta3)*cos(theta4)*sin(theta5)) + 0.1*cos(theta6)*(cos(theta4)*cos(theta6) + cos(theta5)*sin(theta4)*sin(theta6)) + 0.1*sin(theta6)*(cos(theta4)*sin(theta6) - 1.0*cos(theta5)*cos(theta6)*sin(theta4)),                                                                                                                                                                                                                                                                                                                                                                                                                                                                                                                                                                                                                                                                                                                                                                                                                                                                                                                                                                                                                                                                                                                                                                                                                                                                                                                                                                                                                                                                                                                                                                                                                                                                                                                                                                                                                                                                                                                                                                                                                                                                                                                                                                                        0.36*cos(theta4) - 0.32*cos(theta4)*cos(theta6) - 0.16*cos(theta4)*sin(theta5) + 0.16*cos(theta4)*cos(theta6)^2 - 0.16*cos(theta5)*sin(theta4)*sin(theta6) + 0.16*cos(theta4)*cos(theta6)*sin(theta5) + 0.16*cos(theta5)*cos(theta6)*sin(theta4)*sin(theta6),                                                                                                                                                                                                                                                                                                                                                                                                                                                                                                                                                                                                                                                                                                                                                                                                                                                                                                                                                                                                                                                                                                                                                                                                                                                                                                                                                                                                                                                                                                                                                                                                                                                                                                                             -0.4*sin(theta5)*sin(theta6)*(0.4*cos(theta6) - 0.4),                                                                                                                                                                                                                                                                                                                                                                                                                                                                                                                                                                                                                                                                                                                                                                                                                                                                                                                                                                                                                                                                                                                                                                                      0.16*cos(theta6)^2 - 0.32*cos(theta6) + 0.36,                                                                                                                                                                                                                                                                                                                                                                                                                                                                                                                                                                                                                                                                                                                                                                                                           0;
                                                                                                                                                                                                                                                                                                                                                                                                                                                                                                                                                                                                                                                                                                                                                                                                                                                                                                                                                                                                                                                                                                                                                                                                                                                                                                                                                                                                                                                                                                                                                                                                                                                                                                                                                                                                                                                                                                                                                                                                                                                                                                                                                                                                                                                                                                                                                                                                                                                                                                                                                                                                                                                                                                                                                                                                                                                                                                                                                                                                                                                                                                                                                                                                                                                                                                                                                                                                                                                                                                                                                                                                                                                                                                                                                                                                                                                                                                                                                            0.08*cos(theta2)*cos(theta4)*cos(theta6) + 0.26*cos(theta2)*cos(theta5)*sin(theta3) + 0.26*cos(theta3)*cos(theta5)*sin(theta2) + 0.16*cos(theta2)*cos(theta3)*cos(theta4)*cos(theta6) + 0.26*cos(theta2)*cos(theta3)*cos(theta4)*sin(theta5) - 0.16*cos(theta2)*cos(theta5)*cos(theta6)*sin(theta3) - 0.16*cos(theta3)*cos(theta5)*cos(theta6)*sin(theta2) - 0.16*cos(theta4)*cos(theta6)*sin(theta2)*sin(theta3) + 0.08*cos(theta2)*cos(theta5)*sin(theta4)*sin(theta6) - 0.26*cos(theta4)*sin(theta2)*sin(theta3)*sin(theta5) - 0.16*cos(theta2)*cos(theta3)*cos(theta4)*cos(theta6)*sin(theta5) + 0.16*cos(theta2)*cos(theta3)*cos(theta5)*sin(theta4)*sin(theta6) + 0.16*cos(theta4)*cos(theta6)*sin(theta2)*sin(theta3)*sin(theta5) - 0.16*cos(theta5)*sin(theta2)*sin(theta3)*sin(theta4)*sin(theta6),                                                                                                                                                                                                                                                                                                                                                                                                                                                                                                                                                                                                                                                                                                                                                                                                                                                                                                                                                                                                                                                                                                                                                                                                                                                                                                                                                                                                                                                                                                                                                                                                                                                                                                                                                                                                                                                                                                                                                                                                                                                                                                                                                                                                                                                                                                   0.16*cos(theta6)*sin(theta4) + 0.26*sin(theta4)*sin(theta5) - 0.16*cos(theta6)*sin(theta4)*sin(theta5) + 0.08*sin(theta3)*sin(theta5)*sin(theta6) + 0.08*cos(theta3)*cos(theta6)*sin(theta4) - 0.16*cos(theta4)*cos(theta5)*sin(theta6) - 0.08*cos(theta3)*cos(theta4)*cos(theta5)*sin(theta6),                                                                                                                                                                                                                                                                                                                                                                                                                                                                                                                                                                                                                                                                                                                                                                                                                                                                                                                                                                                                                                                                                                                                                                                                                                                                                                                                                                                                                                                                                                                                                                                                                                                                                                                                                                                                                                                                                                                                                                                                                                                                                                                                                                                                                                                                                                   0.16*cos(theta6)*sin(theta4) + 0.26*sin(theta4)*sin(theta5) - 0.16*cos(theta6)*sin(theta4)*sin(theta5) - 0.16*cos(theta4)*cos(theta5)*sin(theta6),                                                                                                                                                                                                                                                                                                                                                                                                                                                                                                                                                                                                                                                                                                                                                                                                                                                                                                                                                                                                                                                                                                                                                                                                                                                                                                                                                                                                                                                                                                                                                                                                                                                                                                                                       -(cos(theta5)*(8.0*cos(theta6) - 13.0))/50,                                                                                                                                                                                                                                                                                                                                                                                                                                                                                                                                                                                                                                                                                                                                                                                                                                                                                                                                                                                                                                                                                                                                                                                                                                 0,                                                                                                                                                                                                                                                                                                                                                                                                                                                                                                                                                                                                                                                                                                                                                                                                        0.26]
 

u=-(MM)*(Ueq+Uas)
u1=u(1);
u2=u(2);
u3=u(3);
u4=u(4);
u5=u(5);
u6=u(6);
